simulink model "SimulinkSimples"  (R2013b)
settings: Solver=ode3  StartTime=0.0  StopTime=20  RelTol=1e-3
settings Model: Creator=ThiagoCordeiro  LastModifiedBy=ThiagoCordeiro

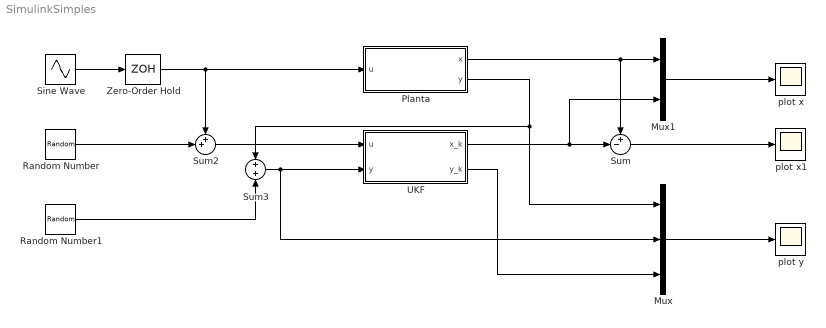
== system SimulinkSimples ==
  Mux : Mux  Inputs=3
  Mux1 : Mux  Inputs=2
  Planta : Subsystem
  Random Number : RandomNumber  Seed=round(rand(1)*(2^32-1))  SampleTime=0.01
  Random Number1 : RandomNumber  Seed=round(rand(1)*(2^32-1))  SampleTime=0.01
  Sine Wave : Sin  Amplitude=2  Phase=pi/2  SampleTime=0
  Sum : Sum  Inputs=+-|
  Sum2 : Sum  Inputs=++|
  Sum3 : Sum  Inputs=+|+
  UKF : Subsystem
  Zero-Order Hold : ZeroOrderHold  SampleTime=0.01
  plot x : Scope
  plot x1 : Scope
  plot y : Scope
      settings: ShowLegends=on  SaveName=ScopeData2
  wires:
  Mux/1 -> plot y/1
  Zero-Order Hold/1 -> Planta/1(u), Sum2/1
  Random Number/1 -> Sum2/2
  Random Number1/1 -> Sum3/2
  Sine Wave/1 -> Zero-Order Hold/1
  Sum2/1 -> UKF/1(u)
  Sum3/1 -> Mux/2, UKF/2(y)
  Planta/2(y) -> Mux/1, Sum3/1
  Planta/1(x) -> Sum/1, Mux1/1
  UKF/1(x_k) -> Sum/2, Mux1/2
  Mux1/1 -> plot x/1
  UKF/2(y_k) -> Mux/3
  Sum/1 -> plot x1/1

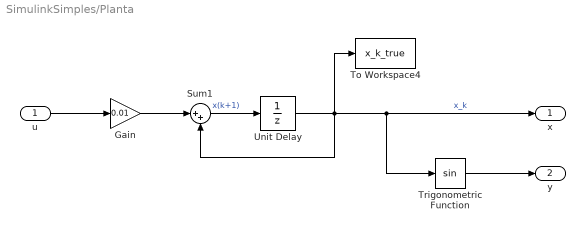
== system SimulinkSimples/Planta ==
  u : Inport
  Gain : Gain  Gain=0.01
  Sum1 : Sum  Inputs=|++
  To Workspace4 : ToWorkspace  VariableName=x_k_true  SampleTime=-1  SaveFormat=Timeseries
  Trigonometric Function : Trigonometry
  Unit Delay : UnitDelay  InitialCondition=[0]  SampleTime=-1
  x : Outport
  y : Outport  Port=2
  wires:
  Sum1/1 -> Unit Delay/1  "x(k+1)"
  Unit Delay/1 -> Sum1/2, Trigonometric Function/1, x/1, To Workspace4/1  "x_k"
  Trigonometric Function/1 -> y/1
  u/1 -> Gain/1
  Gain/1 -> Sum1/1

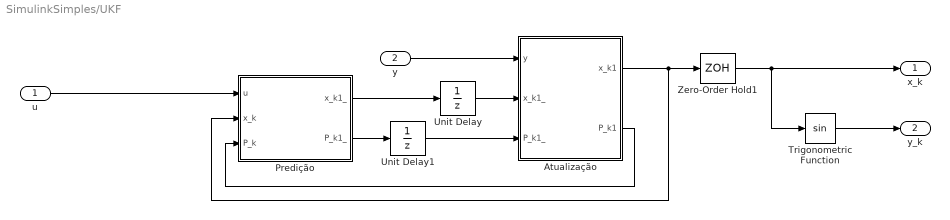
== system SimulinkSimples/UKF ==
  u : Inport
  y : Inport  Port=2
  Atualização : Subsystem
  Predição : Subsystem
  Trigonometric Function : Trigonometry
  Unit Delay : UnitDelay  InitialCondition=randn(1)  SampleTime=0.01
  Unit Delay1 : UnitDelay  InitialCondition=1  SampleTime=0.01
  Zero-Order Hold1 : ZeroOrderHold  SampleTime=0.01
  x_k : Outport
  y_k : Outport  Port=2
  wires:
  u/1 -> Predição/1(u)
  y/1 -> Atualização/1(y)
  Atualização/1(x_k1) -> Predição/2(x_k), Zero-Order Hold1/1
  Atualização/2(P_k1) -> Predição/3(P_k)
  Predição/2(P_k1_) -> Unit Delay1/1
  Unit Delay1/1 -> Atualização/3(P_k1_)
  Unit Delay/1 -> Atualização/2(x_k1_)
  Predição/1(x_k1_) -> Unit Delay/1
  Zero-Order Hold1/1 -> Trigonometric Function/1, x_k/1
  Trigonometric Function/1 -> y_k/1

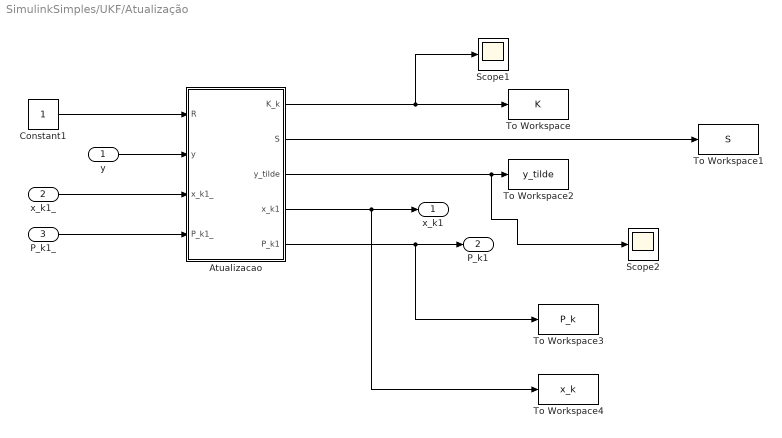
== system SimulinkSimples/UKF/Atualização ==
  y : Inport
  x_k1_ : Inport  Port=2
  P_k1_ : Inport  Port=3
  Atualizacao : MATLAB Function  TreatAsAtomicUnit=on  SystemSampleTime=0.01
  Constant1 : Constant
  Scope1 : Scope
      settings: SaveName=ScopeData3
  Scope2 : Scope
      settings: SaveName=ScopeData5
  To Workspace : ToWorkspace  VariableName=K  SampleTime=-1  SaveFormat=Timeseries
  To Workspace1 : ToWorkspace  VariableName=S  SampleTime=-1  SaveFormat=Timeseries
  To Workspace2 : ToWorkspace  VariableName=y_tilde  SampleTime=-1  SaveFormat=Timeseries
  To Workspace3 : ToWorkspace  VariableName=P_k  SampleTime=-1  SaveFormat=Timeseries
  To Workspace4 : ToWorkspace  VariableName=x_k  SampleTime=-1  SaveFormat=Timeseries
  x_k1 : Outport
  P_k1 : Outport  Port=2
  wires:
  y/1 -> Atualizacao/2(y)
  x_k1_/1 -> Atualizacao/3(x_k1_)
  P_k1_/1 -> Atualizacao/4(P_k1_)
  Atualizacao/4(x_k1) -> To Workspace4/1, x_k1/1
  Atualizacao/5(P_k1) -> To Workspace3/1, P_k1/1
  Constant1/1 -> Atualizacao/1(R)
  Atualizacao/1(K_k) -> Scope1/1, To Workspace/1
  Atualizacao/2(S) -> To Workspace1/1
  Atualizacao/3(y_tilde) -> Scope2/1, To Workspace2/1

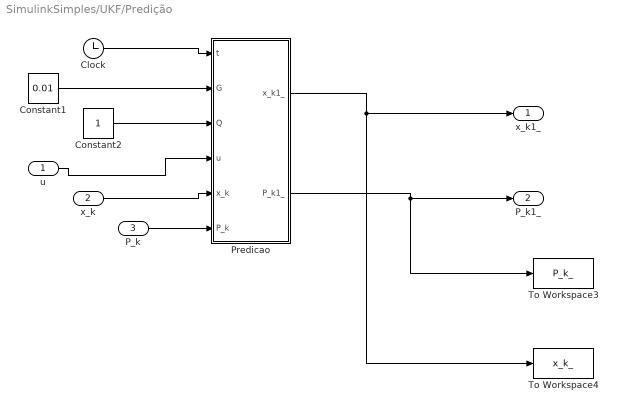
== system SimulinkSimples/UKF/Predição ==
  u : Inport
  x_k : Inport  Port=2
  P_k : Inport  Port=3
  Clock : Clock
  Constant1 : Constant  Value=0.01  VectorParams1D=off
  Constant2 : Constant
  Predicao : MATLAB Function  TreatAsAtomicUnit=on  SystemSampleTime=0.01
  To Workspace3 : ToWorkspace  VariableName=P_k_  SampleTime=-1  SaveFormat=Timeseries
  To Workspace4 : ToWorkspace  VariableName=x_k_  SampleTime=-1  SaveFormat=Timeseries
  x_k1_ : Outport
  P_k1_ : Outport  Port=2
  wires:
  u/1 -> Predicao/4(u)
  x_k/1 -> Predicao/5(x_k)
  P_k/1 -> Predicao/6(P_k)
  Constant1/1 -> Predicao/2(G)
  Constant2/1 -> Predicao/3(Q)
  Predicao/1(x_k1_) -> To Workspace4/1, x_k1_/1
  Predicao/2(P_k1_) -> To Workspace3/1, P_k1_/1
  Clock/1 -> Predicao/1(t)

== matlab function SimulinkSimples/UKF/Atualização/Atualizacao ==
  data: R input; K_k output; S output; y_tilde output; y input; x_k1_ input; P_k1_ input; x_k1 output; P_k1 output
function [K_k, S, y_tilde, x_k1, P_k1] = fcn(R, y, x_k1_, P_k1_)
%#codegen

% Intensidade da dispersão dos pontos
lambda = 1;

n = size(x_k1_,1);
kappa = n + lambda;
peso_1 = lambda/kappa;
peso_2 = 1/(2*kappa);

% gera 2n + 1 sigma points
[X_k, X_k_noMean]  = sigmas(x_k1_,P_k1_,kappa);

Y_k = sensorSig(X_k);
[y_hat, S_semR, Y_k_noMean] = unsTrans(Y_k, [peso_1 peso_2]);
S = S_semR + R;
Pxy = unsCov(X_k_noMean, Y_k_noMean, [peso_1 peso_2]);

K_k  =  Pxy / S;
P_k1 = P_k1_ - K_k * S * K_k';


y_tilde = y - y_hat;
x_k1 = x_k1_ + K_k * y_tilde; 

end

function Y_k = sensorSig(X_k)

nSig = length(X_k);
Y_k_temp = sensorEst(X_k(:,1));
Y_k = zeros(length(Y_k_temp),nSig);
Y_k(:,1) = Y_k_temp;
for ii = 2:nSig
    Y_k(:,ii) = sensorEst(X_k(:,ii));
end    

end

% Funcao possivelmente nao linear da predicao - especifica para cada caso
% Nesse exemplo,a  funcao e linear, e não ha vantagem utilizar UKF
function y_hat = sensorEst(x_k)
y_hat = sin(x_k);
end

== matlab function SimulinkSimples/UKF/Predição/Predicao ==
  data: t input; G input; Q input; u input; x_k1_ output; x_k input; P_k input; P_k1_ output
function [x_k1_,P_k1_] = fcn(t, G, Q, u, x_k, P_k)
%#codegen
if t >= 0
    % Intensidade da dispersão dos pontos
    lambda = 1;
    
    % Matriz Qd - assumida conhecida
    Qd = G*Q*G';
    
    n = size(x_k,1);
    kappa = n + lambda;
    peso_1 = lambda/kappa;
    peso_2 = 1/(2*kappa);
    
    % gera 2n + 1 sigma points
    X_k  = sigmas(x_k,P_k,kappa);
    
    X_k1_ = predSig(X_k, u);
    
    [x_k1_, P_k1_semQ] = unsTrans(X_k1_, [peso_1 peso_2]);
        
    P_k1_ = P_k1_semQ + Qd;
else
    x_k1_ = x_k;
    P_k1_ = P_k;
end

if t > 5
    flag = 1;
end

end

function X_k1_ = predSig(X_k, u)

nSig = length(X_k);
X_k1_ = zeros(size(X_k));
for ii = 1:nSig
    X_k1_(:,ii) = predicao(X_k(:,ii),u);
end    

end

% Funcao possivelmente nao linear da predicao - especifica para cada caso
% Nesse exemplo,a  funcao e linear, e não ha vantagem utilizar UKF
function x_k1_ = predicao(x_k,u)
T = 0.01;

x_k1_ = x_k + T*u;
end
